simulink model "AckermanControl"  (R2023a)
settings: Solver=ode4  StartTime=0.0  StopTime=100  FixedStep=0.01  RelTol=1e-3
InitFcn:
  | params
StopFcn:
  | drawPath
values from neighbouring files (symbols this model uses):
  K = 500    [params.m]
  l = 26    [params.m]
  Ld = 25    [params.m]
  tau = 2    [params.m]
  taud = 0.15    [params.m]
  tauSteer = 0.17    [params.m]
  v = 17    [params.m]
undefined symbols (not defined in the file or in its folder): R, xFine, yFine
libraries: slpidlib x1
settings Model: Creator=AlterraOnix  LastModifiedBy=AlterraOnix

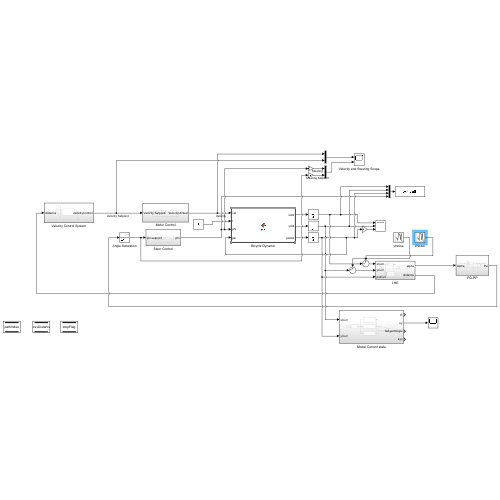
[thumbnail: Simulink's stored preview of the top-level diagram]
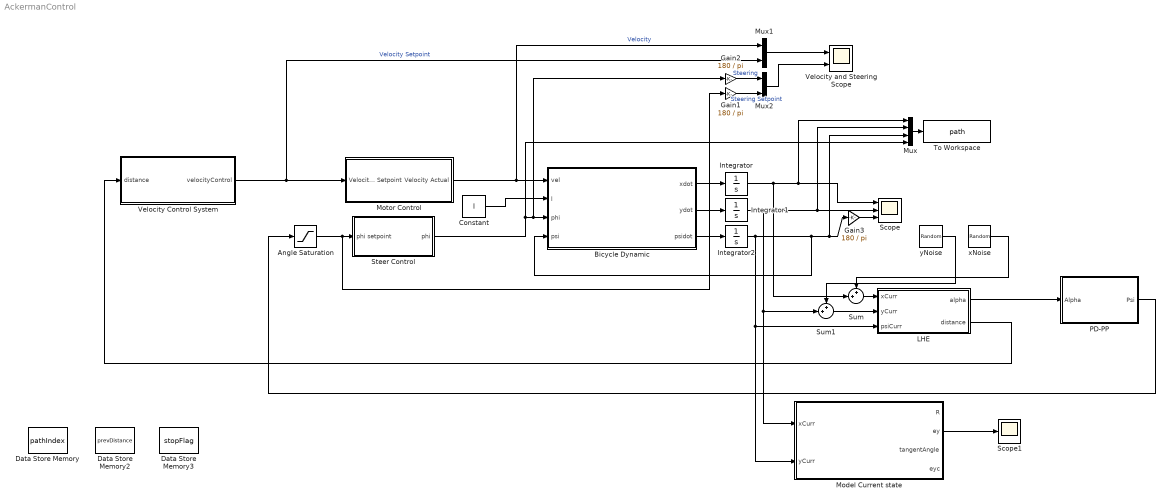
== system AckermanControl ==
  Angle Saturation : Saturate  UpperLimit=30 * pi / 180  LowerLimit=-30 * pi / 180
  Bicycle Dynamic : MATLAB Function  TreatAsAtomicUnit=on
  Constant : Constant  Value=l
  Data Store Memory : DataStoreMemory  DataStoreName=pathIndex  WriteAfterWriteMsg=warning  ShowAdditionalParam=off
  Data Store Memory2 : DataStoreMemory  DataStoreName=prevDistance  WriteAfterWriteMsg=warning  InitialValue=inf  ShowAdditionalParam=off
  Data Store Memory3 : DataStoreMemory  DataStoreName=stopFlag  WriteAfterWriteMsg=warning  ShowAdditionalParam=off
  Gain1 : Gain  Gain=180 / pi
  Gain2 : Gain  Gain=180 / pi
  Gain3 : Gain  Gain=180 / pi
  Integrator : Integrator
  Integrator1 : Integrator  InitialCondition=-15
  Integrator2 : Integrator
  LHE : Subsystem
  Model Current state : Subsystem
  Motor Control : Subsystem
  Mux : Mux
  Mux1 : Mux  Inputs=2
  Mux2 : Mux  Inputs=2
  PD-PP : Subsystem
  Scope : Scope  NumInputPorts=3
  Scope1 : Scope
  Steer Control : Subsystem
  Sum : Sum  Inputs=++|
  Sum1 : Sum  Inputs=++|
  To Workspace : ToWorkspace  VariableName=path  SaveFormat=Timeseries  SampleTime=-1
  Velocity Control System : Subsystem
  Velocity and Steering Scope : Scope  NumInputPorts=2
  xNoise : RandomNumber  Variance=3  Seed=10  SampleTime=0.1
  yNoise : RandomNumber  Variance=3  Seed=10  SampleTime=0.1
  wires:
  Bicycle Dynamic/1(xdot) -> Integrator/1
  Bicycle Dynamic/2(ydot) -> Integrator1/1
  Bicycle Dynamic/3(psidot) -> Integrator2/1
  Integrator1/1 -> Sum1/2, Model Current state/1(xCurr), Mux/2, Scope/2
  Integrator/1 -> Sum/2, Mux/1, Scope/1
  Integrator2/1 -> LHE/3(psiCurr), Model Current state/2(yCurr), Bicycle Dynamic/4(psi), Mux/3, Gain3/1
  Constant/1 -> Bicycle Dynamic/2(l)
  Motor Control/1(Velocity Actual) -> Mux1/1, Bicycle Dynamic/1(vel)  "Velocity"
  Steer Control/1(phi) -> Mux/4, Gain2/1, Bicycle Dynamic/3(phi)
  Gain3/1 -> Scope/3
  Mux/1 -> To Workspace/1
  Velocity Control System/1(velocityControl) -> Motor Control/1(Velocity Setpoint), Mux1/2  "Velocity Setpoint"
  LHE/2(distance) -> Velocity Control System/1(distance)
  Angle Saturation/1 -> Gain1/1, Steer Control/1(phi setpoint)
  Mux2/1 -> Velocity and Steering Scope/2
  LHE/1(alpha) -> PD-PP/1(Alpha)
  PD-PP/1(Psi) -> Angle Saturation/1
  Mux1/1 -> Velocity and Steering Scope/1
  Gain1/1 -> Mux2/2  "Steering Setpoint"
  Gain2/1 -> Mux2/1  "Steering"
  Model Current state/2(ey) -> Scope1/1
  Sum/1 -> LHE/1(xCurr)
  Sum1/1 -> LHE/2(yCurr)
  yNoise/1 -> Sum1/1
  xNoise/1 -> Sum/1

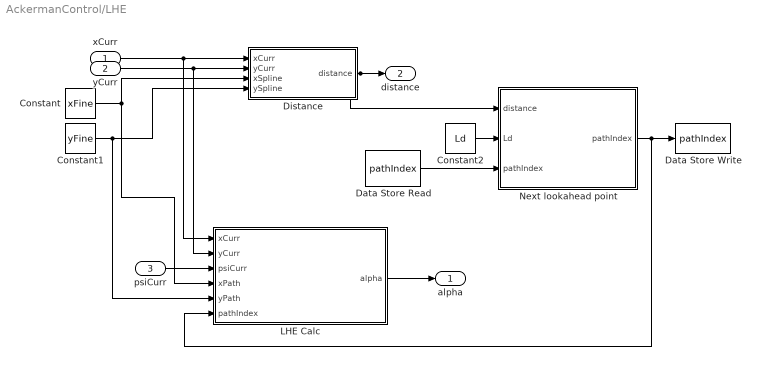
== system AckermanControl/LHE ==
  xCurr : Inport
  yCurr : Inport  Port=2
  psiCurr : Inport  Port=3
  Constant : Constant  Value=xFine
  Constant1 : Constant  Value=yFine
  Constant2 : Constant  Value=Ld
  Data Store Read : DataStoreRead  DataStoreName=pathIndex  IndexOptions=Index vector (dialog)  Indices=1  OutputSizes=1
  Data Store Write : DataStoreWrite  DataStoreName=pathIndex  IndexOptions=Index vector (dialog)  Indices=1  OutputSizes=1
  Distance : MATLAB Function  TreatAsAtomicUnit=on
  LHE Calc : MATLAB Function  TreatAsAtomicUnit=on
  Next lookahead point : MATLAB Function  TreatAsAtomicUnit=on
  alpha : Outport
  distance : Outport  Port=2
  wires:
  xCurr/1 -> LHE Calc/1(xCurr), Distance/1(xCurr)
  yCurr/1 -> LHE Calc/2(yCurr), Distance/2(yCurr)
  Constant/1 -> LHE Calc/4(xPath), Distance/3(xSpline)
  Constant1/1 -> LHE Calc/5(yPath), Distance/4(ySpline)
  Next lookahead point/1(pathIndex) -> LHE Calc/6(pathIndex), Data Store Write/1
  Data Store Read/1 -> Next lookahead point/3("pathIndex ")
  Distance/1(distance) -> Next lookahead point/1(distance), distance/1
  psiCurr/1 -> LHE Calc/3(psiCurr)
  LHE Calc/1(alpha) -> alpha/1
  Constant2/1 -> Next lookahead point/2(Ld)

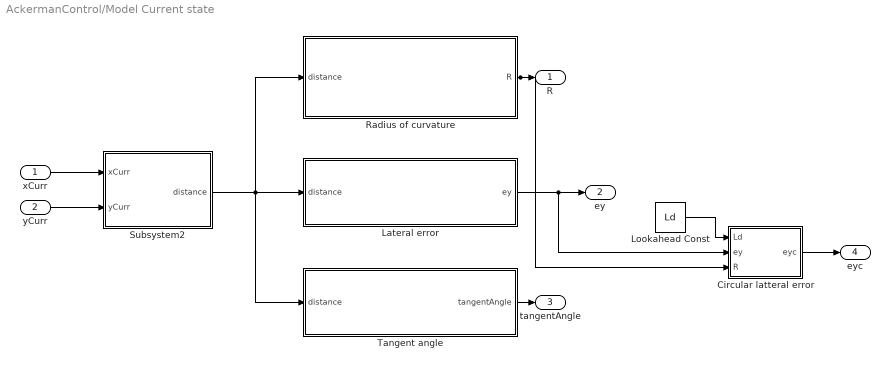
== system AckermanControl/Model Current state ==
  xCurr : Inport
  yCurr : Inport  Port=2
  Circular latteral error : MATLAB Function  TreatAsAtomicUnit=on
  Lateral error : Subsystem
  Lookahead Const : Constant  Value=Ld
  Radius of curvature : Subsystem
  Subsystem2 : Subsystem
  Tangent angle : Subsystem
  R : Outport
  ey : Outport  Port=2
  tangentAngle : Outport  Port=3
  eyc : Outport  Port=4
  wires:
  Radius of curvature/1(R) -> Circular latteral error/3(R), R/1
  Tangent angle/1(tangentAngle) -> tangentAngle/1
  Subsystem2/1(distance) -> Radius of curvature/1(distance), Lateral error/1(distance), Tangent angle/1(distance)
  xCurr/1 -> Subsystem2/1(xCurr)
  yCurr/1 -> Subsystem2/2(yCurr)
  Lateral error/1(ey) -> Circular latteral error/2(ey), ey/1
  Lookahead Const/1 -> Circular latteral error/1(Ld)
  Circular latteral error/1(eyc) -> eyc/1

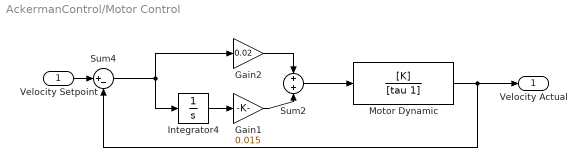
== system AckermanControl/Motor Control ==
  Velocity Setpoint : Inport
  Gain1 : Gain  Gain=0.015
  Gain2 : Gain  Gain=0.02
  Integrator4 : Integrator
  Motor Dynamic : TransferFcn  Numerator=[K]  Denominator=[tau 1]
  Sum2 : Sum
  Sum4 : Sum  Inputs=|+-
  Velocity Actual : Outport
  wires:
  Integrator4/1 -> Gain1/1
  Gain1/1 -> Sum2/2
  Gain2/1 -> Sum2/1
  Motor Dynamic/1 -> Velocity Actual/1, Sum4/2
  Sum4/1 -> Integrator4/1, Gain2/1
  Velocity Setpoint/1 -> Sum4/1
  Sum2/1 -> Motor Dynamic/1

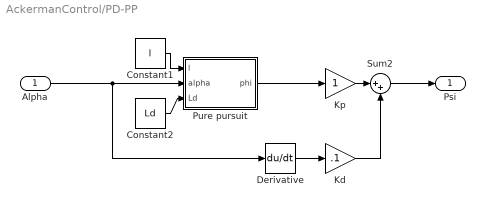
== system AckermanControl/PD-PP ==
  Alpha : Inport
  Constant1 : Constant  Value=l
  Constant2 : Constant  Value=Ld
  Derivative : Derivative
  Kd : Gain  Gain=.1
  Kp : Gain
  Pure pursuit : MATLAB Function  TreatAsAtomicUnit=on
  Sum2 : Sum  Inputs=|++
  Psi : Outport
  wires:
  Pure pursuit/1(phi) -> Kp/1
  Constant2/1 -> Pure pursuit/3(Ld)
  Kd/1 -> Sum2/2
  Constant1/1 -> Pure pursuit/1(l)
  Sum2/1 -> Psi/1
  Derivative/1 -> Kd/1
  Kp/1 -> Sum2/1
  Alpha/1 -> Derivative/1, Pure pursuit/2(alpha)

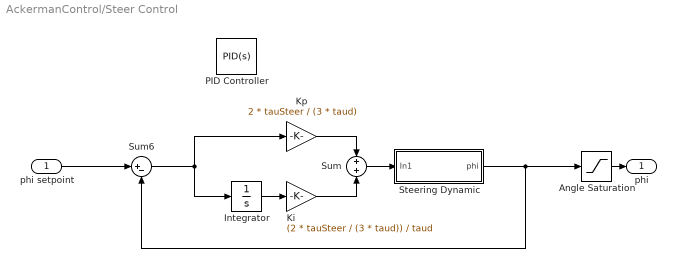
== system AckermanControl/Steer Control ==
  phi setpoint : Inport
  Angle Saturation : Saturate  UpperLimit=30 * pi / 180  LowerLimit=-30 * pi / 180
  Integrator : Integrator
  Ki : Gain  Gain=(2 * tauSteer / (3 * taud)) / taud
  Kp : Gain  Gain=2 * tauSteer / (3 * taud)
  PID Controller : slpidlib/PID Controller  Controller=PID  Form=Parallel  TimeDomain=Continuous-time  UseExternalTs=off  SampleTime=-1  IntegratorMethod=Forward Euler  FilterMethod=Forward Euler  ControllerParametersSource=internal  P=2 * tauSteer / (3 * taud)  I=(2 * tauSteer / (3 * taud)) / taud  UseKiTs=off  D=0  N=100  UseFilter=on  TunerSelectOption=Transfer Function Based (PID Tuner App)  InitialConditionSource=internal  InitialConditionForIntegrator=0  InitialConditionForFilter=0  DifferentiatorICPrevScaledInput=0  ExternalReset=none  TrackingMode=off  Kt=1  LimitOutput=off  SatLimitsSource=internal  UpperSaturationLimit=inf  LowerSaturationLimit=-inf  LinearizeAsGain=on  AntiWindupMode=none  Kb=1  LimitIntegrator=off  UpperIntegratorSaturationLimit=inf  LowerIntegratorSaturationLimit=-inf  POutMin=[]  POutMax=[]  IOutMin=[]  IOutMax=[]  DOutMin=[]  DOutMax=[]  NOutMin=[]  NOutMax=[]  SumOutMin=[]  SumOutMax=[]  SaturationOutMin=[]  SaturationOutMax=[]  PParamMin=[]  PParamMax=[]  IParamMin=[]  IParamMax=[]  DParamMin=[]  DParamMax=[]  NParamMin=[]  NParamMax=[]  KbParamMin=[]  KbParamMax=[]  KtParamMin=[]  KtParamMax=[]  KbOutMin=[]  KbOutMax=[]  KtOutMin=[]  KtOutMax=[]  IntegratorOutMin=[]  IntegratorOutMax=[]  FilterOutMin=[]  FilterOutMax=[]  SumI1OutMin=[]  SumI1OutMax=[]  SumI2OutMin=[]  SumI2OutMax=[]  SumI3OutMin=[]  SumI3OutMax=[]  SumI4OutMin=[]  SumI4OutMax=[]  SumDOutMin=[]  SumDOutMax=[]  DifferentiatorOutMin=[]  DifferentiatorOutMax=[]  FilterDiffOutCoefMin=[]  FilterDiffOutCoefMax=[]  ReciprocalOutMin=[]  ReciprocalOutMax=[]  SumDenOutMin=[]  SumDenOutMax=[]  SumNumOutMin=[]  SumNumOutMax=[]  DivideOutMin=[]  DivideOutMax=[]  UdiffTsProdOutMin=[]  UdiffTsProdOutMax=[]  NTsProdOutMin=[]  NTsProdOutMax=[]  UintegralTsProdOutMin=[]  UintegralTsProdOutMax=[]  UngainTsProdOutMin=[]  UngainTsProdOutMax=[]  ClampingZeroOutDataTypeStr=Inherit: Inherit via back propagation  ClampingZeroOutMin=[]  ClampingZeroOutMax=[]  FilterDenConstantOutDataTypeStr=Inherit: Inherit via back propagation  FilterDenConstantOutMin=[]  FilterDenConstantOutMax=[]  PCopyOutDataTypeStr=Inherit: Inherit via back propagation  PCopyOutMin=[]  PCopyOutMax=[]  NCopyOutDataTypeStr=Inherit: Inherit via back propagation  NCopyOutMin=[]  NCopyOutMax=[]  IntegratorContinuousStateAttributes=''  IntegratorStateMustResolveToSignalObject=off  IntegratorRTWStateStorageClass=Auto  FilterContinuousStateAttributes=''  FilterStateMustResolveToSignalObject=off  FilterRTWStateStorageClass=Auto  ParallelPVariant=InternalParameters  IdealPVariant=Disabled  IVariant=InternalParameters  DVariant=InternalParameters  IntegratorVariant=Continuous  SatVariant=Disabled  AWVariant=Passthrough  PCopyVariant=Disabled  TRVariant=Disabled  FdbkBlocksVariant=Forward  IdealPFdbkVariant=Disabled  SatFdbkVariant=Disabled  DerivativeFilterVariant=ContFilter  NVariant=InternalParameters  NCopyVariant=Disabled  FilterICVariant=InternalICsFilter  IntegratorICVariant=InternalICs  ExternalResetVariant=Disabled  TRSumVariant=Passthrough  SumFdbkVariant=Disabled  SumVariant=Sum_PID  TsampFilterVariant=InternalTs  TsampNgainVariant=Passthrough  TsampIntegralVariant=Disabled_SignalSpec  ExternalSaturationOutDataTypeStr=Inherit: Same as second input
  Steering Dynamic : Subsystem
  Sum : Sum
  Sum6 : Sum  Inputs=|+-
  phi : Outport
  wires:
  Steering Dynamic/1(phi) -> Angle Saturation/1, Sum6/2
  phi setpoint/1 -> Sum6/1
  Sum/1 -> Steering Dynamic/1(In1)
  Kp/1 -> Sum/1
  Sum6/1 -> Integrator/1, Kp/1
  Integrator/1 -> Ki/1
  Ki/1 -> Sum/2
  Angle Saturation/1 -> phi/1

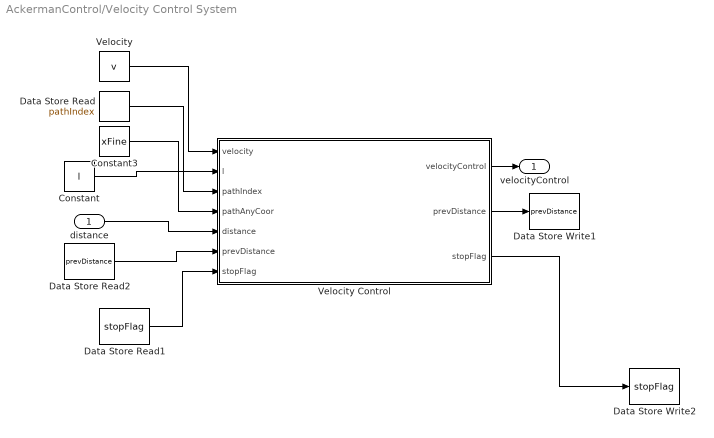
== system AckermanControl/Velocity Control System ==
  distance : Inport
  Constant : Constant  Value=l
  Constant3 : Constant  Value=xFine
  Data Store Read : DataStoreRead  DataStoreName=pathIndex  IndexOptions=Index vector (dialog)  Indices=1  OutputSizes=1
  Data Store Read1 : DataStoreRead  DataStoreName=stopFlag  IndexOptions=Index vector (dialog)  Indices=1  OutputSizes=1
  Data Store Read2 : DataStoreRead  DataStoreName=prevDistance  IndexOptions=Index vector (dialog)  Indices=1  OutputSizes=1
  Data Store Write1 : DataStoreWrite  DataStoreName=prevDistance  IndexOptions=Index vector (dialog)  Indices=1  OutputSizes=1
  Data Store Write2 : DataStoreWrite  DataStoreName=stopFlag  IndexOptions=Index vector (dialog)  Indices=1  OutputSizes=1
  Velocity : Constant  Value=v
  Velocity Control : MATLAB Function  TreatAsAtomicUnit=on
  velocityControl : Outport
  wires:
  Constant3/1 -> Velocity Control/4(pathAnyCoor)
  Velocity/1 -> Velocity Control/1(velocity)
  Data Store Read2/1 -> Velocity Control/6("prevDistance ")
  Velocity Control/2(prevDistance) -> Data Store Write1/1
  Data Store Read/1 -> Velocity Control/3(pathIndex)
  distance/1 -> Velocity Control/5(distance)
  Velocity Control/1(velocityControl) -> velocityControl/1
  Data Store Read1/1 -> Velocity Control/7("stopFlag ")
  Velocity Control/3(stopFlag) -> Data Store Write2/1
  Constant/1 -> Velocity Control/2(l)

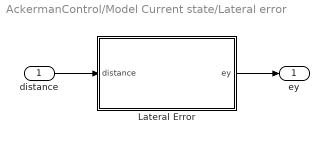
== system AckermanControl/Model Current state/Lateral error ==
  distance : Inport
  Lateral Error : MATLAB Function  TreatAsAtomicUnit=on
  ey : Outport
  wires:
  Lateral Error/1(ey) -> ey/1
  distance/1 -> Lateral Error/1(distance)

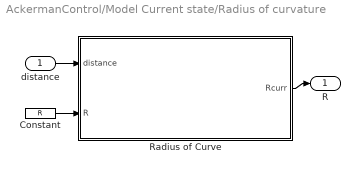
== system AckermanControl/Model Current state/Radius of curvature ==
  distance : Inport
  Constant : Constant  Value=R
  Radius of Curve : MATLAB Function  TreatAsAtomicUnit=on
  R : Outport
  wires:
  distance/1 -> Radius of Curve/1(distance)
  Radius of Curve/1(Rcurr) -> R/1
  Constant/1 -> Radius of Curve/2(R)

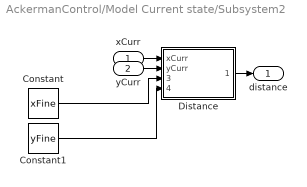
== system AckermanControl/Model Current state/Subsystem2 ==
  xCurr : Inport
  yCurr : Inport  Port=2
  Constant : Constant  Value=xFine
  Constant1 : Constant  Value=yFine
  Distance : MATLAB Function  TreatAsAtomicUnit=on
  distance : Outport
  wires:
  xCurr/1 -> Distance/1(xCurr)
  yCurr/1 -> Distance/2(yCurr)
  Distance/1(distance) -> distance/1
  Constant/1 -> Distance/3(xSpline)
  Constant1/1 -> Distance/4(ySpline)

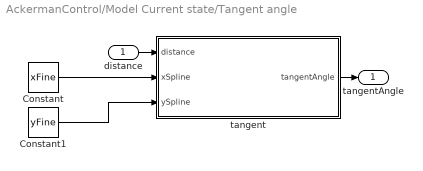
== system AckermanControl/Model Current state/Tangent angle ==
  distance : Inport
  Constant : Constant  Value=xFine
  Constant1 : Constant  Value=yFine
  tangent : MATLAB Function  TreatAsAtomicUnit=on
  tangentAngle : Outport
  wires:
  tangent/1(tangentAngle) -> tangentAngle/1
  distance/1 -> tangent/1(distance)
  Constant/1 -> tangent/2(xSpline)
  Constant1/1 -> tangent/3(ySpline)

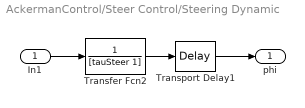
== system AckermanControl/Steer Control/Steering Dynamic ==
  In1 : Inport
  Transfer Fcn2 : TransferFcn  Denominator=[tauSteer 1]
  Transport Delay1 : TransportDelay  DelayTime=taud
  phi : Outport
  wires:
  Transport Delay1/1 -> phi/1
  Transfer Fcn2/1 -> Transport Delay1/1
  In1/1 -> Transfer Fcn2/1

== matlab function AckermanControl/Velocity Control System/Velocity Control ==
  data: velocity input; l input; velocityControl output; pathIndex input; pathAnyCoor input; distance input; prevDistance output; prevDistance input; stopFlag input; stopFlag output
function [velocityControl, prevDistance, stopFlag] = fcn(velocity, l, pathIndex, pathAnyCoor, distance, prevDistance, stopFlag)
    if pathIndex >= size(pathAnyCoor)
        if ((distance(end) < 15)) || stopFlag == 1
            velocityControl = 0;
            prevDistance = 0; % Ensure stopping
            stopFlag = 1;
        else
            velocityControl = velocity;
            prevDistance = distance(end);
        end
    else
        velocityControl = velocity;
        prevDistance = distance(end);
    end

== matlab function AckermanControl/Model Current state/Circular latteral error ==
  data: Ld input; eyc output; ey input; R input
function eyc = fcn(Ld, ey, R)
    eyc = (-Ld^2 - ey^2 + 2 * R * ey) / (2 * (R - ey));

== matlab function AckermanControl/Model Current state/Radius of curvature/Radius of Curve ==
  data: distance input; Rcurr output; R input
function Rcurr = fcn(distance, R)
    
    [~, minIdx] = min(distance);

    Rcurr = R(minIdx);

== matlab function AckermanControl/Bicycle Dynamic ==
  data: vel input; xdot output; l input; phi input; ydot output; psidot output; psi input
function [xdot, ydot, psidot] = fcn(vel, l, phi, psi)
    matrix = [cos(psi)      0               0
              0             sin(psi)        0
              0             0               tan(phi)];

    lengthVector = [1; 1; 1 / l];
    globalVel = matrix * lengthVector * vel;
    xdot = globalVel(1);
    ydot = globalVel(2);
    psidot = globalVel(3);

== matlab function AckermanControl/Model Current state/Lateral error/Lateral Error ==
  data: distance input; ey output
function ey = fcn(distance)
    [ey, ~] = min(distance);

== matlab function AckermanControl/Model Current state/Tangent angle/tangent ==
  data: distance input; tangentAngle output; xSpline input; ySpline input
function tangentAngle = fcn(distance, xSpline, ySpline)
    [~, idx] = min(distance);
    
    step = 2;
    if idx <= step
        dy = ySpline(idx + step) - ySpline(idx);
        dx = xSpline(idx + step) - xSpline(idx);
    elseif idx >= length(xSpline) - step
        dy = ySpline(idx) - ySpline(idx - step);
        dx = xSpline(idx) - xSpline(idx - step);
    else 
        dy = ySpline(idx + step) - ySpline(idx - step);
        dx = xSpline(idx + step) - xSpline(idx - step);
    end

    tangentAngle = atan2(dy, dx);

== matlab function AckermanControl/Model Current state/Subsystem2/Distance ==
  data: xCurr input; distance output; yCurr input; xSpline input; ySpline input
function distance = fcn(xCurr, yCurr, xSpline, ySpline)
    distance = sqrt((xSpline - xCurr) .^ 2 + (ySpline - yCurr) .^ 2);

== matlab function AckermanControl/LHE/LHE Calc ==
  data: xCurr input; alpha output; yCurr input; psiCurr input; xPath input; yPath input; pathIndex input
function alpha = fcn(xCurr, yCurr, psiCurr, xPath, yPath, pathIndex)
    dy = yPath(pathIndex) - yCurr;
    dx = xPath(pathIndex) - xCurr;

    % instead of geometric calculation and using if else, just rotate the
    % points
    rotMat = [cos(psiCurr)  sin(psiCurr)
              -sin(psiCurr)  cos(psiCurr)];

    rotatedPointDiff = rotMat * [dx; dy];
    alpha = atan2(rotatedPointDiff(2), rotatedPointDiff(1));

== matlab function AckermanControl/LHE/Next lookahead point ==
  data: distance input; pathIndex output; Ld input; pathIndex input
function pathIndex  = fcn(distance, Ld, pathIndex)
    [~, minPathIdx] = mink(abs(distance - Ld), 2);
    for idx = 1: 2
        if minPathIdx(idx) > pathIndex && minPathIdx(idx) < pathIndex + 100
            pathIndex = minPathIdx(idx);
            break
        end
    end

== matlab function AckermanControl/LHE/Distance ==
  data: xCurr input; distance output; yCurr input; xSpline input; ySpline input
function distance = fcn(xCurr, yCurr, xSpline, ySpline)
    distance = sqrt((xSpline - xCurr) .^ 2 + (ySpline - yCurr) .^ 2);

== matlab function AckermanControl/PD-PP/Pure pursuit ==
  data: l input; phi output; alpha input; Ld input
function phi = fcn(l, alpha, Ld)
    phi = 2 * l * alpha / Ld;
